simulink model "dspsdadc4"  (Simulink 7.4)
settings: Solver=ode45  SolverMode=SingleTasking  StartTime=0.0  StopTime=inf  FixedStep=1/512000  MaxStep=1e-6  RelTol=1e-3  AbsTol=1e-6
libraries: dspmlti4 x3, simulink x1, dspsnks4 x1, dspobslib x1
settings Model: Creator=don  LastModifiedBy=Dick  ExtModeTrigMode=oneshot  ExtModeArmWhenConnect=off
settings DataIOCC: LimitDataPoints=off  SaveOutput=off  SaveTime=off  SignalLoggingName=sigsOut
settings OptimizationCC: BlockReduction=off  BooleanDataType=off  InitFltsAndDblsToZero=on
settings DebuggingCC: SaveWithParameterizedLinksMsg=none  SignalResolutionControl=TryResolveAllWithWarning  SolverPrmCheckMsg=none  MultiTaskDSMMsg=warning  MultiTaskCondExecSysMsg=none  IntegerOverflowMsg=none  StrictBusMsg=None
settings HardwareCC: TargetUnknown=on
settings RTWCC: IncludeERTFirstTime=on
settings GRTTargetCC: TargetFcnLib=ansi_tfl_tmw.mat

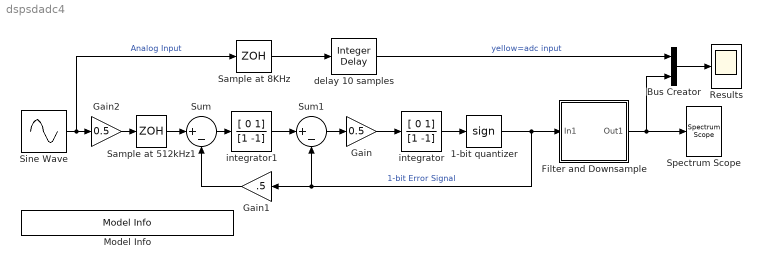
== system dspsdadc4 ==
  1-bit quantizer : Signum
  Bus Creator : BusCreator  Inputs=2
  Filter and Downsample : Subsystem
  Gain : Gain  Gain=0.5  ParameterDataType=sfix(16)  ParameterScaling=2^0  OutDataType=sfix(16)  OutScaling=2^0  SaturateOnIntegerOverflow=on  OutDataTypeStr=Inherit: Same as input  ParamDataTypeStr=Inherit: Same as input
  Gain1 : Gain  Gain=.5  ParameterDataType=sfix(16)  ParameterScaling=2^0  OutDataType=sfix(16)  OutScaling=2^0  SaturateOnIntegerOverflow=on  OutDataTypeStr=Inherit: Same as input  ParamDataTypeStr=Inherit: Same as input
  Gain2 : Gain  Gain=0.5  ParameterDataType=sfix(16)  ParameterScaling=2^0  OutDataType=sfix(16)  OutScaling=2^0  SaturateOnIntegerOverflow=on  OutDataTypeStr=Inherit: Same as input  ParamDataTypeStr=Inherit: Same as input
  Model Info : simulink/Model-Wide Utilities/Model Info  SystemSampleTime=-1  InitialBlockCM=none  BlockCM=none  Frame=on  DisplayStringWithTags=Copywrite 2005-2010 The MathWorks, Inc.  HorizontalTextAlignment=Center  LeftAlignmentValue=0.5  SourceBlockDiagram=dspsdadc4  TagMaxNumber=20
  Results : Scope
      settings: TimeRange=0.015  YMin=-1  YMax=1  DataFormat=Array
  Sample at 512kHz1 : ZeroOrderHold  SampleTime=1/512000
  Sample at 8KHz : ZeroOrderHold  SampleTime=1/8000
  Sine Wave : Sin  Amplitude=.5  Bias=0  Frequency=500*2*pi  Phase=0  Samples=10  SampleTime=0  Offset=0
  Spectrum Scope : dspsnks4/Spectrum Scope  DialogController=dspdialog.SpectrumScope  DialogControllerArgs=DataTag3  SystemSampleTime=-1  ScopeProperties=off  Domain=Frequency  HorizSpan=1  UseBuffer=on  BufferSize=512  Overlap=0  inpFftLenInherit=off  FFTlength=128  numAvg=1  DisplayProperties=off  AxisGrid=on  Memory=off  FrameNumber=on  AxisLegend=off  AxisZoom=off  OpenScopeAtSimStart=on  OpenScopeImmediately=off  FigPos=[4 36 640 268]  AxisProperties=on  XUnits=Hertz  XRange=[0...Fs/2]  XDisplay=0  InheritXIncr=on  XIncr=1.0  XLabel=Samples  XLimit=Auto  YUnits=dB  XMax=1  XMin=0  YLabel=Magnitude, dB  LineProperties=off  wintypeSpecScope=Hann  RsSpecScope=50  betaSpecScope=5  winsampSpecScope=Periodic  XAxisParamsVer=6.8
      settings: YMin=-80  YMax=20
  Sum : Sum  Inputs=|+-  OutDataType=sfix(16)  OutScaling=2^0  SaturateOnIntegerOverflow=on  InputSameDT=on  OutDataTypeStr=Inherit: Same as first input
  Sum1 : Sum  Inputs=|+-  OutDataType=sfix(16)  OutScaling=2^0  SaturateOnIntegerOverflow=on  InputSameDT=on  OutDataTypeStr=Inherit: Same as first input
  delay 10 samples : dspobslib/Integer Delay  delay=10  ic=0  reset_popup=None
  integrator : DiscreteFilter  Numerator=[ 0 1]  Denominator=[1 -1]
  integrator1 : DiscreteFilter  Numerator=[ 0 1]  Denominator=[1 -1]
  wires:
  Filter and Downsample/1(Out1) -> Bus Creator/2, Spectrum Scope/1
  Sine Wave/1 -> Gain2/1, Sample at 8KHz/1  "Analog Input"
  1-bit quantizer/1 -> Filter and Downsample/1(In1), Sum1/2, Gain1/1  "1-bit Error Signal"
  Sum/1 -> integrator1/1
  Bus Creator/1 -> Results/1
  Sample at 8KHz/1 -> delay 10 samples/1
  delay 10 samples/1 -> Bus Creator/1  "yellow=adc input"
  integrator1/1 -> Sum1/1
  Sum1/1 -> Gain/1
  Gain/1 -> integrator/1
  Gain1/1 -> Sum/2
  Sample at 512kHz1/1 -> Sum/1
  integrator/1 -> 1-bit quantizer/1
  Gain2/1 -> Sample at 512kHz1/1

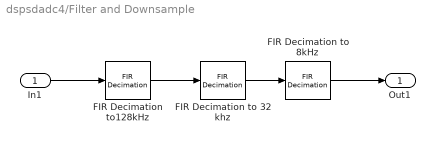
== system dspsdadc4/Filter and Downsample ==
  In1 : Inport  OutDataType=sfix(16)  OutScaling=2^0
  FIR Decimation to 32 khz : dspmlti4/FIR Decimation  DialogController=dspdialog.FIRDecimation  DialogControllerArgs=DataTag0  h=fir1(64, 0.1)  D=4  filtStruct=Direct form  framing=Maintain input frame size  outputBufInitCond=0  roundingMode=Floor  overflowMode=off  FilterSource=Specify via dialog  FilterObject=Hm_firdecim
  FIR Decimation to 8kHz : dspmlti4/FIR Decimation  DialogController=dspdialog.FIRDecimation  DialogControllerArgs=DataTag1  h=fir1(64, 0.075)  D=4  filtStruct=Direct form  framing=Maintain input frame size  outputBufInitCond=0  roundingMode=Floor  overflowMode=off  FilterSource=Specify via dialog  FilterObject=Hm_firdecim
  FIR Decimation to128kHz : dspmlti4/FIR Decimation  DialogController=dspdialog.FIRDecimation  DialogControllerArgs=DataTag2  h=fir1(64, 0.125)  D=4  filtStruct=Direct form  framing=Maintain input frame size  outputBufInitCond=0  roundingMode=Floor  overflowMode=off  FilterSource=Specify via dialog  FilterObject=Hm_firdecim
  Out1 : Outport  OutDataType=sfix(16)  OutScaling=2^0
  wires:
  FIR Decimation to 32 khz/1 -> FIR Decimation to 8kHz/1
  FIR Decimation to128kHz/1 -> FIR Decimation to 32 khz/1
  In1/1 -> FIR Decimation to128kHz/1
  FIR Decimation to 8kHz/1 -> Out1/1
